simulink model "testemplanner_cs"  (R2023a)
settings: Solver=ode5  StartTime=0.0  StopTime=70  FixedStep=1/1000  RelTol=1e-3
PreLoadFcn:
  | mbxruntime.callbacks.PreLoadFcn(bdroot);
PostLoadFcn:
  | mbxruntime.callbacks.PostLoadFcn(bdroot);
InitFcn:
  | mbxruntime.callbacks.InitFcn(bdroot);
StartFcn:
  | mbxruntime.callbacks.StartFcn(bdroot);
StopFcn:
  | mbxruntime.callbacks.StopFcn(bdroot);
model workspace (MAT data in the model file):
  mbox_table : object (value not decoded)
  model_closed = 0
  sim_status = 0
values from neighbouring files (symbols this model uses):
  c_factor = 43.75    [emplanner_init.m]
  cf = -175016    [emplanner_init.m]
  cr = -130634    [emplanner_init.m]
  global_path_x = [-4.4795 -3.48011774493 -2.48199463442 -1.48514775065 -0.489582877207 0.504698358082 1.49769585569 2.48941007764 3.47984169183 4.46899144113 5.45686009523 6.44344843293 ... (3001 elements, 3001x1)]    [global_path.mat]
  global_path_y = [6.0531 6.0531 6.0531 6.0531 6.0531 6.0531 6.0531 6.0531 6.0531 6.0531 6.0531 6.0531 ... (3001 elements, 3001x1)]    [global_path.mat]
  KD_PID_distance = 0.0    (= 0)    [emplanner_init.m]
  KD_PID_speed = 0    [emplanner_init.m]
  KI_PID_distance = 0.0    (= 0)    [emplanner_init.m]
  KI_PID_speed = 0    [emplanner_init.m]
  KP_PID_distance = 0.5    [emplanner_init.m]
  KP_PID_speed = 1.8    [emplanner_init.m]
  la = 1.265    [emplanner_init.m]
  lb = 2.947-1.265    (= 1.682)    [emplanner_init.m]
  LQR_K1 = k(:,1)'    [emplanner_init.m]
  LQR_K2 = k(:,2)'    [emplanner_init.m]
  LQR_K3 = k(:,3)'    [emplanner_init.m]
  LQR_K4 = k(:,4)'    [emplanner_init.m]
  m = 2020    [emplanner_init.m]
  rack_displacement = [-39.14 , -37.2 , -35.29 , -33.43 , -31.6 , -29.81 , -28.06 , -26.34 , -24.66 ,      -23.01 , -21.38 , -19.79 , -18.23 , -16.69 , -15.18 , -13.7 , -12.23 , -10.8 , -9.38 , -7.98 ,     -6.61 , -5.25 , -3.91 , -2.59 , -1.29 , 0 , 1.27 , 2.54 , 3.78 , 5.02 , 6.24 , 7.46 , 8.66 ,      9.86 , 11.05 , 12.24 , 13.41 , 14.59 , 15.76 , 16.92 , 18.09 , 19.25 , 20.42 , 21.59 , 22.76 ,      23.93 , 25.11 , 26 ...(+26 chars)    [emplanner_init.m]
  right_wheel_ground = [-70 ,-67.2 , -64.4 , -61.6 , -58.8 , -56 , -53.2 , -50.4 , -47.6 , -44.8 , -42 ,      -39.2 , -36.4 , -33.6 , -30.8 , -28 , -25.2 , -22.4 , -19.6 , -16.8 , -14 , -11.2 , -8.4 , -5.6 ,      -2.8 , 0 , 2.8 , 5.6 , 8.4 , 11.2 , 14 , 16.8 , 19.6 , 22.4 , 25.2 , 28 , 30.8 , 33.6 , 36.4 ,      39.2 , 42 , 44.8 , 47.6 , 50.4 , 53.2 , 56 , 58.8 , 61.6 , 64.4 , 67.2 , 70 ]    [emplanner_init.m]
  vx_break_point = zeros(1,5000)    [emplanner_init.m]
undefined symbols (not defined in the file or in its folder): aubr, DiscIntNeverNeededParam, tablebr, vubr, warningInitialVelocity, x0
libraries: PreScanSimulinkLibrary x19, simulink x19, simulink_extras x6, Solver_SF x1
(part 4 of 10)

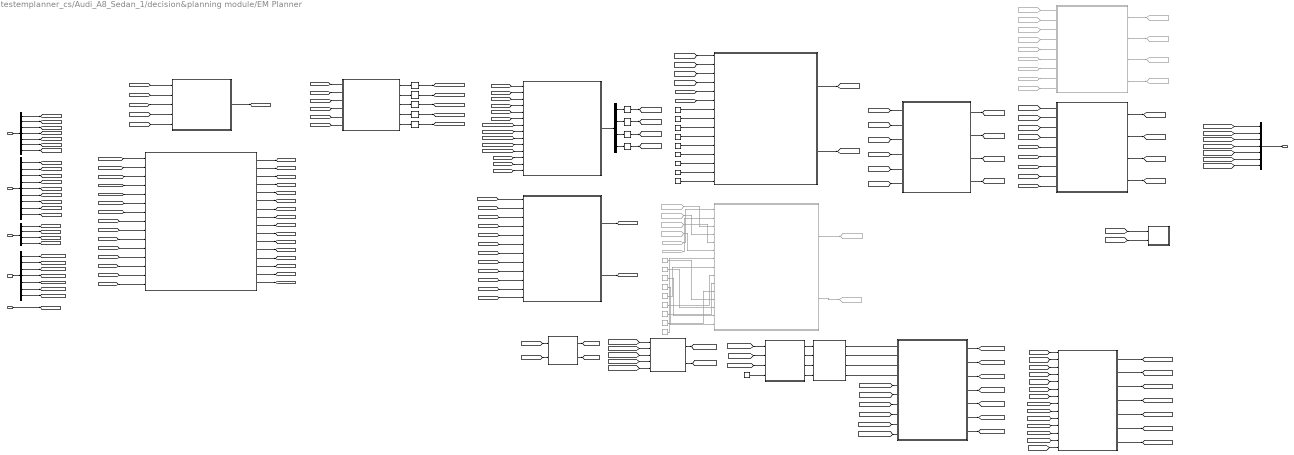
== system testemplanner_cs/Audi_A8_Sedan_1/decision&planning module/EM Planner ==
  referenceline_info : Inport
  location_info : Inport  Port=2
  perception_info : Inport  Port=3
  pre_planning_info : Inport  Port=4
  current time : Inport  Port=5
  Bus Creator : BusCreator  Inputs=7
  Bus Selector : BusSelector  OutputSignals=referenceline_x,referenceline_y,referenceline_heading,referenceline_kappa,origin_match_point_index,origin_proj_x,origin_proj_y
  Bus Selector1 : BusSelector  OutputSignals=host_x,host_y,host_heading_xy,host_vx,host_vy,host_yawrate,host_speed,host_ax,host_ay
  Bus Selector2 : BusSelector  OutputSignals=obs_x_set_gcs,obs_y_set_gcs,obs_velocity_set_gcs,obs_heading_set_gcs
  Bus Selector3 : BusSelector  OutputSignals=trajectory_x_gcs,trajectory_y_gcs,trajectory_heading_gcs,trajectory_kappa_gcs,trajectory_speed_gcs,trajectory_accel_gcs,trajectory_time_gcs
  Bus Selector4 : BusSelector  OutputSignals=s_set,l_set,dl_set,ddl_set
  Cartesian2Frenet-panning start point : Subsystem
  Constant : Constant  Value=9
  Constant1 : Constant  Value=4
  Constant10 : Constant  Commented=on  Value=9
  Constant11 : Constant  Commented=on  Value=4
  Constant12 : Constant  Commented=on  Value=15
  Constant13 : Constant  Commented=on
  Constant14 : Constant  Commented=on  Value=300
  Constant15 : Constant  Commented=on  Value=2000
  Constant16 : Constant  Commented=on  Value=10000
  Constant17 : Constant  Commented=on  Value=20
  Constant18 : Constant  Commented=on  Value=1e8
  Constant2 : Constant  Value=15
  Constant3 : Constant
  Constant4 : Constant  Value=300
  Constant5 : Constant  Value=2000
  Constant6 : Constant  Value=10000
  Constant7 : Constant  Value=20
  Constant8 : Constant  Value=1e8
  Constant9 : Constant  Value=8
  Dynamic Programming : MATLAB Function  TreatAsAtomicUnit=on
  Frenet2Cartesian : MATLAB Function  TreatAsAtomicUnit=on
  Frenet2Cartesian1 : MATLAB Function  Commented=on  TreatAsAtomicUnit=on
  From103 : From  Commented=on  GotoTag=planning_start_dl
  From109 : From  Commented=on  GotoTag=planning_start_ddl
  From116 : From  Commented=on  GotoTag=static_obs_s_set
  From117 : From  Commented=on  GotoTag=static_obs_l_set
  From118 : From  Commented=on  GotoTag=dp_path_s_final
  From119 : From  Commented=on  GotoTag=dp_path_l_final
  From120 : From  Commented=on  GotoTag=dp_path_dl_final
  From121 : From  Commented=on  GotoTag=dp_path_ddl_final
  From122 : From  Commented=on  GotoTag=referenceline_x
  From123 : From  Commented=on  GotoTag=referenceline_y
  From124 : From  Commented=on  GotoTag=referenceline_heading
  From125 : From  Commented=on  GotoTag=referenceline_kappa
  From126 : From  Commented=on  GotoTag=index2s
  From92 : From  Commented=on  GotoTag=planning_start_s
  From93 : From  Commented=on  GotoTag=planning_start_l
  Goto66 : Goto  Commented=on  GotoTag=dp_path_s_init
  Goto67 : Goto  Commented=on  GotoTag=dp_path_l_init
  Goto86 : Goto  Commented=on  GotoTag=trajectory_x_init
  Goto87 : Goto  Commented=on  GotoTag=trajectory_y_init
  Goto88 : Goto  Commented=on  GotoTag=trajectory_heading_init
  Goto89 : Goto  Commented=on  GotoTag=trajectory_kappa_init
  MATLAB Function : MATLAB Function  TreatAsAtomicUnit=on
  MATLAB Function1 : MATLAB Function  TreatAsAtomicUnit=on
  Obs : Subsystem
  Selector{1..9} (9 alike) : Selector  InputPortWidth=128  IndexOptions=Index vector (dialog)  Indices=1  OutputSizes=1
  cacul planning start gcs : MATLAB Function  TreatAsAtomicUnit=on
  calc path length and map between point and s : MATLAB Function  TreatAsAtomicUnit=on
  calc speed planning start condition : MATLAB Function  TreatAsAtomicUnit=on
  generate index2s : MATLAB Function  TreatAsAtomicUnit=on
  increase st point count : MATLAB Function  TreatAsAtomicUnit=on
  match&proj point search2 : MATLAB Function  TreatAsAtomicUnit=on
  path and speed merge : MATLAB Function  TreatAsAtomicUnit=on
  path decision with dynamic planning(dp) : MATLAB Function  Commented=on  TreatAsAtomicUnit=on
  simple speed qp planning : MATLAB Function  TreatAsAtomicUnit=on
  stitch trajectory : MATLAB Function  TreatAsAtomicUnit=on
  EM Planner result : Outport
  wires:
  referenceline_info/1 -> Bus Selector/1
  Bus Selector/1 -> [referenceline_x]  "<referenceline_x>"
  Bus Selector/2 -> [referenceline_y]  "<referenceline_y>"
  Bus Selector/3 -> [referenceline_heading]  "<referenceline_heading>"
  Bus Selector/4 -> [referenceline_kappa]  "<referenceline_kappa>"
  location_info/1 -> Bus Selector1/1
  Bus Selector1/1 -> [host_x]  "<host_x>"
  Bus Selector1/2 -> [host_y]  "<host_y>"
  Bus Selector1/3 -> [host_heading_xy]  "<host_heading_xy>"
  Bus Selector1/4 -> [host_vx_vcs]  "<host_vx>"
  Bus Selector1/5 -> [host_vy_vcs]  "<host_vy>"
  Bus Selector1/6 -> [host_yawrate]  "<host_yawrate>"
  Bus Selector1/7 -> [host_speed]  "<host_speed>"
  Bus Selector1/8 -> [host_ax_vcs]  "<host_ax>"
  Bus Selector1/9 -> [host_ay_vcs]  "<host_ay>"
  perception_info/1 -> Bus Selector2/1
  Bus Selector2/1 -> [obs_x_set_gcs]  "<obs_x_set_gcs>"
  Bus Selector2/2 -> [obs_y_set_gcs]  "<obs_y_set_gcs>"
  Bus Selector2/3 -> [obs_velocity_set_gcs]  "<obs_velocity_set_gcs>"
  Bus Selector2/4 -> [obs_heading_set_gcs]  "<obs_heading_set_gcs>"
  pre_planning_info/1 -> Bus Selector3/1
  Bus Selector3/1 -> [pre_trajectory_x_gcs]  "<trajectory_x_gcs>"
  Bus Selector3/2 -> [pre_trajectory_y_gcs]  "<trajectory_y_gcs>"
  Bus Selector3/3 -> [pre_trajectory_heading_gcs]  "<trajectory_heading_gcs>"
  Bus Selector3/4 -> [pre_trajectory_kappa_gcs]  "<trajectory_kappa_gcs>"
  Bus Selector3/5 -> [pre_trajectory_speed_gcs]  "<trajectory_speed_gcs>"
  Bus Selector3/6 -> [pre_trajectory_accel_gcs]  "<trajectory_accel_gcs>"
  current time/1 -> [current_time]
  [pre_trajectory_x_gcs] -> cacul planning start gcs/1(pre_trajectory_x)
  [pre_trajectory_y_gcs] -> cacul planning start gcs/2(pre_trajectory_y)
  [pre_trajectory_heading_gcs] -> cacul planning start gcs/3(pre_trajectory_heading)
  [pre_trajectory_kappa_gcs] -> cacul planning start gcs/4(pre_trajectory_kappa)
  [pre_trajectory_speed_gcs] -> cacul planning start gcs/5(pre_trajectory_speed)
  [pre_trajectory_accel_gcs] -> cacul planning start gcs/6(pre_trajectory_accel)
  [pre_trajectory_time] -> cacul planning start gcs/7(pre_trajectory_time)
  [current_time] -> cacul planning start gcs/8(current_time)
  [host_x] -> cacul planning start gcs/9(host_x)
  [host_y] -> cacul planning start gcs/10(host_y)
  [host_heading_xy] -> cacul planning start gcs/11(host_heading_xy)
  [host_vx_vcs] -> cacul planning start gcs/12(host_vx)
  [host_vy_vcs] -> cacul planning start gcs/13(host_vy)
  [host_ax_vcs] -> cacul planning start gcs/14(host_ax)
  [host_ay_vcs] -> cacul planning start gcs/15(host_ay)
  cacul planning start gcs/1(planning_start_x) -> [planning_start_x]
  cacul planning start gcs/2(planning_start_y) -> [planning_start_y]
  cacul planning start gcs/3(planning_start_heading) -> [planning_start_heading]
  cacul planning start gcs/4(planning_start_kappa) -> [planning_start_kappa]
  cacul planning start gcs/5(planning_start_vx) -> [planning_start_vx]
  cacul planning start gcs/6(planning_start_vy) -> [planning_start_vy]
  cacul planning start gcs/7(planning_start_ax) -> [planning_start_ax]
  cacul planning start gcs/8(planning_start_ay) -> [planning_start_ay]
  cacul planning start gcs/9(planning_start_time) -> [planning_start_time]
  cacul planning start gcs/10(stitch_x) -> [stitch_x]
  cacul planning start gcs/11(stitch_y) -> [stitch_y]
  cacul planning start gcs/12(stitch_heading) -> [stitch_heading]
  cacul planning start gcs/13(stitch_kappa) -> [stitch_kappa]
  cacul planning start gcs/14(stitch_speed) -> [stitch_speed]
  cacul planning start gcs/15(stitch_accel) -> [stitch_accel]
  cacul planning start gcs/16(stitch_time) -> [stitch_time]
  Bus Selector/5 -> [origin_match_point_index]  "<origin_match_point_index>"
  Bus Selector/6 -> [origin_proj_x]  "<origin_proj_x>"
  Bus Selector/7 -> [origin_proj_y]  "<origin_proj_y>"
  [origin_match_point_index] -> generate index2s/1(origin_match_point_index)
  [origin_proj_x] -> generate index2s/2(origin_proj_x)
  [origin_proj_y] -> generate index2s/3(origin_proj_y)
  [referenceline_x] -> generate index2s/4(path_x)
  [referenceline_y] -> generate index2s/5(path_y)
  generate index2s/1(index2s) -> [index2s]
  match&proj point search2/3(proj_y_set) -> Selector3/1
  match&proj point search2/1(match_point_index_set) -> Selector1/1
  match&proj point search2/2(proj_x_set) -> Selector2/1
  match&proj point search2/4(proj_heading_set) -> Selector4/1
  match&proj point search2/5(proj_kappa_set) -> Selector5/1
  [planning_start_x] -> match&proj point search2/1(x_set)
  [planning_start_y] -> match&proj point search2/2(y_set)
  [referenceline_x] -> match&proj point search2/3(frenet_x_set)
  [referenceline_y] -> match&proj point search2/4(frenet_y_set)
  [referenceline_heading] -> match&proj point search2/5(frenet_heading_set)
  [referenceline_kappa] -> match&proj point search2/6(frenet_kapppa_set)
  Selector1/1 -> [planning_start_match_point_index]
  Selector2/1 -> [planning_start_proj_x]
  Selector3/1 -> [planning_start_proj_y]
  Selector4/1 -> [planning_start_proj_heading]
  Selector5/1 -> [planning_start_proj_kappa]
  Cartesian2Frenet-panning start point/1(Caetesian2Frenetout) -> Bus Selector4/1
  Bus Selector4/1 -> Selector6/1  "<s_set>"
  Bus Selector4/2 -> Selector7/1  "<l_set>"
  Bus Selector4/3 -> Selector8/1  "<dl_set>"
  Bus Selector4/4 -> Selector9/1  "<ddl_set>"
  [planning_start_x] -> Cartesian2Frenet-panning start point/1(x_set)
  [planning_start_y] -> Cartesian2Frenet-panning start point/2(y_set)
  [planning_start_vx] -> Cartesian2Frenet-panning start point/3(vx_set)
  [planning_start_vy] -> Cartesian2Frenet-panning start point/4(vy_set)
  [planning_start_ax] -> Cartesian2Frenet-panning start point/5(ax_set)
  [planning_start_ay] -> Cartesian2Frenet-panning start point/6(ay_set)
  [planning_start_proj_x] -> Cartesian2Frenet-panning start point/7(proj_x_set)
  [planning_start_proj_y] -> Cartesian2Frenet-panning start point/8(proj_y_set)
  [planning_start_proj_heading] -> Cartesian2Frenet-panning start point/9(proj_heading_set)
  [planning_start_proj_kappa] -> Cartesian2Frenet-panning start point/10(proj_kappa_set)
  [planning_start_match_point_index] -> Cartesian2Frenet-panning start point/11(match_point_index_set)
  [referenceline_x] -> Cartesian2Frenet-panning start point/12(frenet_x_set)
  [referenceline_y] -> Cartesian2Frenet-panning start point/13(frenet_y_set)
  [index2s] -> Cartesian2Frenet-panning start point/14(index2s)
  Selector6/1 -> [planning_start_s]
  Selector7/1 -> [planning_start_l]
  Selector8/1 -> [planning_start_dl]
  Selector9/1 -> [planning_start_ddl]
  [host_x] -> Obs/1(host_x)
  [host_y] -> Obs/2(host_y)
  [obs_x_set_gcs] -> Obs/3(obs_x_set_gcs)
  [obs_y_set_gcs] -> Obs/4(obs_y_set_gcs)
  [obs_velocity_set_gcs] -> Obs/5(obs_velocity_set_gcs)
  [obs_heading_set_gcs] -> Obs/6(obs_heading_set_gcs)
  [host_heading_xy] -> Obs/7(host_heading_xy)
  [index2s] -> Obs/12(index2s)
  [referenceline_x] -> Obs/8(referenceline_x)
  [referenceline_y] -> Obs/9(referenceline_y)
  [referenceline_heading] -> Obs/10(referenceline_heading)
  [referenceline_kappa] -> Obs/11(referenceline_kappa)
  Obs/1(static_obs_s_set) -> [static_obs_s_set]
  Obs/2(static_obs_l_set) -> [static_obs_l_set]
  [planning_start_s] -> Dynamic Programming/1(planning_start_s)
  [planning_start_l] -> Dynamic Programming/2(planning_start_l)
  [planning_start_dl] -> Dynamic Programming/3(planning_start_dl)
  [planning_start_ddl] -> Dynamic Programming/4(planning_start_ddl)
  [static_obs_l_set] -> Dynamic Programming/6(obs_l_set)
  [static_obs_s_set] -> Dynamic Programming/5(obs_s_set)
  Constant/1 -> Dynamic Programming/7(row)
  Constant1/1 -> Dynamic Programming/8(col)
  Constant2/1 -> Dynamic Programming/9(sample_s)
  Constant3/1 -> Dynamic Programming/10(sample_l)
  Constant4/1 -> Dynamic Programming/11(w_dl_smooth_cost)
  Constant5/1 -> Dynamic Programming/12(w_ddl_smooth_cost)
  Constant6/1 -> Dynamic Programming/13(w_dddl_smooth_cost)
  Constant7/1 -> Dynamic Programming/14(w_reference_cost)
  Constant8/1 -> Dynamic Programming/15(w_collision_cost)
  Dynamic Programming/1(dp_path_s) -> [dp_path_s_init]
  Dynamic Programming/2(dp_path_l) -> [dp_path_l_init]
  [dp_path_s_init] -> MATLAB Function/1(dp_path_s_init)
  [dp_path_l_init] -> MATLAB Function/2(dp_path_l_init)
  [planning_start_s] -> MATLAB Function/3(plan_start_s)
  [planning_start_dl] -> MATLAB Function/5(plan_start_dl)
  [planning_start_ddl] -> MATLAB Function/6(plan_start_ddl)
  [planning_start_l] -> MATLAB Function/4(plan_start_l)
  MATLAB Function/1(dp_path_s_final) -> [dp_path_s_final]
  MATLAB Function/2(dp_path_l_final) -> [dp_path_l_final]
  MATLAB Function/3(dp_path_dl_final) -> [dp_path_dl_final]
  MATLAB Function/4(dp_path_ddl_final) -> [dp_path_ddl_final]
  [dp_path_s_final] -> Frenet2Cartesian/1(s_set)
  [dp_path_l_final] -> Frenet2Cartesian/2(l_set)
  [dp_path_dl_final] -> Frenet2Cartesian/3(dl_set)
  [dp_path_ddl_final] -> Frenet2Cartesian/4(ddl_set)
  [referenceline_x] -> Frenet2Cartesian/5(frenet_x)
  [referenceline_y] -> Frenet2Cartesian/6(frenet_y)
  [referenceline_heading] -> Frenet2Cartesian/7(frenet_heading)
  [index2s] -> Frenet2Cartesian/9(index2s)
  [referenceline_kappa] -> Frenet2Cartesian/8(frenet_kappa)
  Frenet2Cartesian/1(x_point_set) -> [trajectory_x_init]
  Frenet2Cartesian/2(y_point_set) -> [trajectory_y_init]
  Frenet2Cartesian/3(heading_point_set) -> [trajectory_heading_init]
  Frenet2Cartesian/4(kappa_point_set) -> [trajectory_kappa_init]
  stitch trajectory/6(trajectory_accel_final) -> [trajectory_accel_final]
  stitch trajectory/7(trajectory_time_final) -> [trajectory_time_final]
  [trajectory_heading] -> stitch trajectory/3(trajectory_heading)
  [planning_start_time] -> path and speed merge/5(current_time)
  increase st point count/2(s_dot) -> path and speed merge/2(s_dot)
  [plan_start_s_dot] -> simple speed qp planning/1(plan_start_s_dot)
  [trajectory_x_final] -> Bus Creator/1  "trajectory_x_gcs"
  [stitch_kappa] -> stitch trajectory/11(stitch_kappa)
  [trajectory_y_final] -> Bus Creator/2  "trajectory_y_gcs"
  simple speed qp planning/4(relative_time_init) -> increase st point count/4(relative_time_init)
  path and speed merge/5(trajectory_speed) -> [trajectory_speed]
  simple speed qp planning/3(s_dot2_init) -> increase st point count/3(s_dot2_init)
  increase st point count/4(relative_time) -> path and speed merge/4(relative_time)
  [plan_start_s_dot2] -> simple speed qp planning/2(plan_start_s_dot2)
  simple speed qp planning/1(s_init) -> increase st point count/1(s_init)
  [trajectory_heading_init] -> path and speed merge/9(trajectory_heading_init)
  path and speed merge/7(trajectory_time) -> [trajectory_time]
  [trajectory_x] -> stitch trajectory/1(trajectory_x)
  path and speed merge/6(trajectory_accel) -> [trajectory_accel]
  [stitch_speed] -> stitch trajectory/12(stitch_speed)
  [trajectory_y] -> stitch trajectory/2(trajectory_y)
  [stitch_accel] -> stitch trajectory/13(stitch_accel)
  stitch trajectory/3(trajectory_heading_final) -> [trajectory_heading_final]
  [trajectory_x_init] -> path and speed merge/7(trajectory_x_init)
  [path_s] -> path and speed merge/6(path_s)
  [path_s_end] -> simple speed qp planning/3(s_end)
  calc speed planning start condition/2(plan_start_s_dot2) -> [plan_start_s_dot2]
  stitch trajectory/5(trajectory_speed_final) -> [trajectory_speed_final]
  Constant9/1 -> simple speed qp planning/4(recommend_T)
  [trajectory_time] -> stitch trajectory/7(trajectory_time)
  [stitch_time] -> stitch trajectory/14(stitch_time)
  [planning_start_ay] -> calc speed planning start condition/4(plan_start_ay)
  [trajectory_accel] -> stitch trajectory/6(trajectory_accel)
  [stitch_heading] -> stitch trajectory/10(stitch_heading)
  [trajectory_kappa] -> stitch trajectory/4(trajectory_kappa)
  [trajectory_heading_final] -> Bus Creator/3  "trajectory_heading_gcs"
  [trajectory_speed_final] -> Bus Creator/5  "trajectory_speed_gcs"
  increase st point count/3(s_dot2) -> path and speed merge/3(s_dot2)
  calc path length and map between point and s/2(path_s) -> [path_s]
  [trajectory_time_final] -> Bus Creator/7  "trajectory_time_gcs"
  stitch trajectory/4(trajectory_kappa_final) -> [trajectory_kappa_final]
  calc path length and map between point and s/1(path_s_end) -> [path_s_end]
  [planning_start_vy] -> calc speed planning start condition/2(plan_start_vy)
  increase st point count/1(s) -> path and speed merge/1(s)
  [planning_start_heading] -> calc speed planning start condition/5(plan_start_heading)
  [trajectory_accel_final] -> Bus Creator/6  "trajectory_accel_gcs"
  path and speed merge/4(trajectory_kappa) -> [trajectory_kappa]
  [stitch_y] -> stitch trajectory/9(stitch_y)
  path and speed merge/1(trajectory_x) -> [trajectory_x]
  stitch trajectory/1(trajectory_x_final) -> [trajectory_x_final]
  [trajectory_x_init] -> calc path length and map between point and s/1(trajectory_x)
  stitch trajectory/2(trajectory_y_final) -> [trajectory_y_final]
  calc speed planning start condition/1(plan_start_s_dot) -> [plan_start_s_dot]
  [trajectory_y_init] -> calc path length and map between point and s/2(trajectory_y)
  [trajectory_speed] -> stitch trajectory/5(trajectory_speed)
  [trajectory_kappa_init] -> path and speed merge/10(trajectory_kappa_init)
  [planning_start_vx] -> calc speed planning start condition/1(plan_start_vx)
  [trajectory_y_init] -> path and speed merge/8(trajectory_y_init)
  path and speed merge/2(trajectory_y) -> [trajectory_y]
  path and speed merge/3(trajectory_heading) -> [trajectory_heading]
  Bus Creator/1 -> EM Planner result/1
  [stitch_x] -> stitch trajectory/8(stitch_x)
  simple speed qp planning/2(s_dot_init) -> increase st point count/2(s_dot_init)
  [planning_start_ax] -> calc speed planning start condition/3(plan_start_ax)
  [trajectory_kappa_final] -> Bus Creator/4  "trajectory_kappa_gcs"
  Bus Selector3/7 -> [pre_trajectory_time]  "<trajectory_time_gcs>"
  [dp_path_s_final] -> MATLAB Function1/1(s)
  [dp_path_l_final] -> MATLAB Function1/2(l)
  path decision with dynamic planning(dp)/2(dp_path_l) -> Goto67/1
  path decision with dynamic planning(dp)/1(dp_path_s) -> Goto66/1
  Constant18/1 -> path decision with dynamic planning(dp)/7(w_cost_collision)
  Constant17/1 -> path decision with dynamic planning(dp)/11(w_cost_ref)
  Constant16/1 -> path decision with dynamic planning(dp)/10(w_cost_smooth_dddl)
  Constant15/1 -> path decision with dynamic planning(dp)/9(w_cost_smooth_ddl)
  Constant14/1 -> path decision with dynamic planning(dp)/8(w_cost_smooth_dl)
  Constant13/1 -> path decision with dynamic planning(dp)/15(sample_l)
  Constant12/1 -> path decision with dynamic planning(dp)/14(sample_s)
  Constant11/1 -> path decision with dynamic planning(dp)/13(col)
  Constant10/1 -> path decision with dynamic planning(dp)/12(row)
  From116/1 -> path decision with dynamic planning(dp)/1(obs_s_set)
  From117/1 -> path decision with dynamic planning(dp)/2(obs_l_set)
  From109/1 -> path decision with dynamic planning(dp)/6(plan_start_dll)
  From103/1 -> path decision with dynamic planning(dp)/5(plan_start_dl)
  From93/1 -> path decision with dynamic planning(dp)/4(plan_start_l)
  From92/1 -> path decision with dynamic planning(dp)/3(plan_start_s)
  Frenet2Cartesian1/4(kappa_set) -> Goto89/1
  Frenet2Cartesian1/3(heading_set) -> Goto88/1
  Frenet2Cartesian1/2(y_set) -> Goto87/1
  Frenet2Cartesian1/1(x_set) -> Goto86/1
  From125/1 -> Frenet2Cartesian1/8(frenet_path_kappa)
  From126/1 -> Frenet2Cartesian1/9(index2s)
  From124/1 -> Frenet2Cartesian1/7(frenet_path_heading)
  From123/1 -> Frenet2Cartesian1/6(frenet_path_y)
  From122/1 -> Frenet2Cartesian1/5(frenet_path_x)
  From121/1 -> Frenet2Cartesian1/4(ddl_set)
  From120/1 -> Frenet2Cartesian1/3(dl_set)
  From119/1 -> Frenet2Cartesian1/2(l_set)
  From118/1 -> Frenet2Cartesian1/1(s_set)

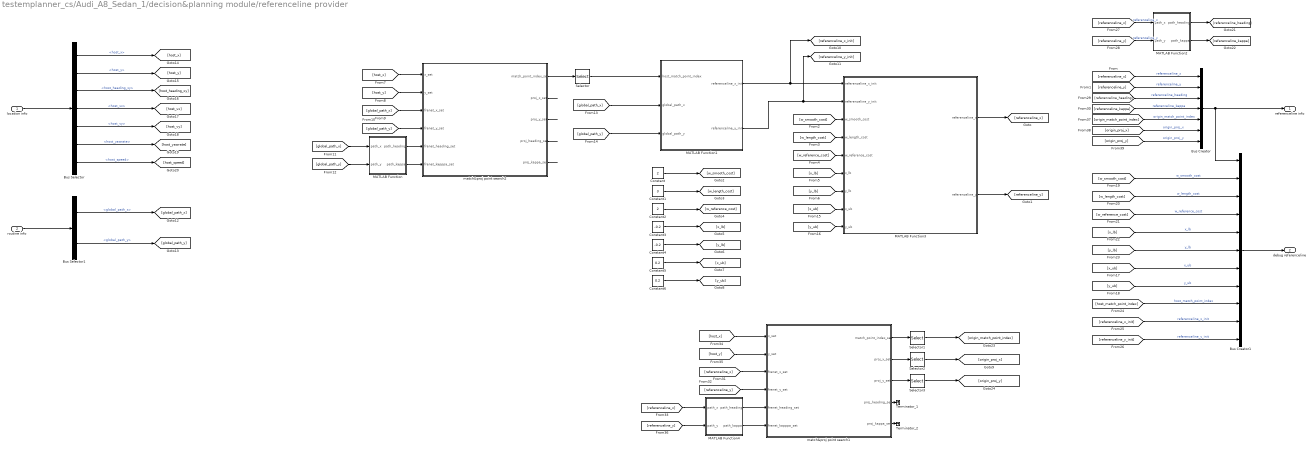
== system testemplanner_cs/Audi_A8_Sedan_1/decision&planning module/referenceline provider ==
  location info : Inport
  routine info : Inport  Port=2
  Bus Creator : BusCreator  Inputs=7
  Bus Creator1 : BusCreator  Inputs=11
  Bus Selector : BusSelector  OutputSignals=host_x,host_y,host_heading_xy,host_vx,host_vy,host_yawrate,host_speed
  Bus Selector1 : BusSelector  OutputSignals=global_path_x,global_path_y
  Constant : Constant  Value=2
  Constant1 : Constant  Value=3
  Constant2 : Constant  Value=2
  Constant3 : Constant  Value=-0.2
  Constant4 : Constant  Value=-0.2
  Constant5 : Constant  Value=0.2
  Constant6 : Constant  Value=0.2
  MATLAB Function : MATLAB Function  TreatAsAtomicUnit=on
  MATLAB Function1 : MATLAB Function  TreatAsAtomicUnit=on
  MATLAB Function2 : MATLAB Function  TreatAsAtomicUnit=on
  MATLAB Function3 : MATLAB Function  TreatAsAtomicUnit=on
  MATLAB Function4 : MATLAB Function  TreatAsAtomicUnit=on
  Selector{,1..3} (4 alike) : Selector  InputPortWidth=128  IndexOptions=Index vector (dialog)  Indices=1  OutputSizes=1
  Terminator_1 : Terminator
  Terminator_2 : Terminator
  match&proj point search1 : MATLAB Function  TreatAsAtomicUnit=on
  match&proj point search2 : MATLAB Function  TreatAsAtomicUnit=on
  referenceline info : Outport
  debug referenceline : Outport  Port=2
  wires:
  [x_lb] -> MATLAB Function3/6(x_lb)
  [global_path_x] -> MATLAB Function/1(path_x)
  [global_path_x] -> match&proj point search2/3(frenet_x_set)
  [w_reference_cost] -> MATLAB Function3/5(w_reference_cost)
  MATLAB Function1/1(referenceline_x_init) -> [referenceline_x_init], MATLAB Function3/1(referenceline_x_init)
  [w_smooth_cost] -> MATLAB Function3/3(w_smooth_cost)
  [host_y] -> match&proj point search2/2(y_set)
  match&proj point search2/1(match_point_index_set) -> Selector/1
  [global_path_y] -> MATLAB Function/2(path_y)
  MATLAB Function/2(path_kappa) -> match&proj point search2/6(frenet_kapppa_set)
  Constant4/1 -> [y_lb]
  [global_path_x] -> MATLAB Function1/2(global_path_x)
  MATLAB Function/1(path_heading) -> match&proj point search2/5(frenet_heading_set)
  [global_path_y] -> MATLAB Function1/3(global_path_y)
  Selector/1 -> MATLAB Function1/1(host_match_point_index)
  Constant2/1 -> [w_reference_cost]
  [global_path_y] -> match&proj point search2/4(frenet_y_set)
  [host_x] -> match&proj point search2/1(x_set)
  [w_length_cost] -> MATLAB Function3/4(w_length_cost)
  MATLAB Function1/2(referenceline_y_init) -> [referenceline_y_init], MATLAB Function3/2(referenceline_y_init)
  Constant/1 -> [w_smooth_cost]
  Constant1/1 -> [w_length_cost]
  Constant3/1 -> [x_lb]
  [x_ub] -> MATLAB Function3/8(x_ub)
  [y_lb] -> MATLAB Function3/7(y_lb)
  [y_ub] -> MATLAB Function3/9(y_ub)
  Constant6/1 -> [y_ub]
  Constant5/1 -> [x_ub]
  MATLAB Function3/1(referenceline_x) -> [referenceline_x]
  MATLAB Function3/2(referenceline_y) -> [referenceline_y]
  Bus Creator/1 -> Bus Creator1/1, referenceline info/1
  [referenceline_y] -> Bus Creator/2  "referenceline_y"
  [referenceline_x] -> Bus Creator/1  "referenceline_x"
  Bus Creator1/1 -> debug referenceline/1
  [w_smooth_cost] -> Bus Creator1/2  "w_smooth_cost"
  [w_length_cost] -> Bus Creator1/3  "w_length_cost"
  [w_reference_cost] -> Bus Creator1/4  "w_reference_cost"
  [x_lb] -> Bus Creator1/5  "x_lb"
  [y_lb] -> Bus Creator1/6  "y_lb"
  [x_ub] -> Bus Creator1/7  "x_ub"
  [y_ub] -> Bus Creator1/8  "y_ub"
  [host_match_point_index] -> Bus Creator1/9  "host_match_point_index"
  [referenceline_x_init] -> Bus Creator1/10  "referenceline_x_init"
  [referenceline_y_init] -> Bus Creator1/11  "referenceline_y_init"
  Bus Selector1/2 -> [global_path_y]  "<global_path_y>"
  Bus Selector1/1 -> [global_path_x]  "<global_path_x>"
  routine info/1 -> Bus Selector1/1
  Bus Selector/7 -> [host_speed]  "<host_speed>"
  Bus Selector/6 -> [host_yawrate]  "<host_yawrate>"
  Bus Selector/2 -> [host_y]  "<host_y>"
  Bus Selector/1 -> [host_x]  "<host_x>"
  Bus Selector/3 -> [host_heading_xy]  "<host_heading_xy>"
  Bus Selector/4 -> [host_vx]  "<host_vx>"
  Bus Selector/5 -> [host_vy]  "<host_vy>"
  location info/1 -> Bus Selector/1
  [referenceline_y] -> MATLAB Function2/2(path_y)  "referenceline_y"
  [referenceline_x] -> MATLAB Function2/1(path_x)  "referenceline_x"
  MATLAB Function2/1(path_heading) -> [referenceline_heading]
  MATLAB Function2/2(path_kappa) -> [referenceline_kappa]
  [referenceline_heading] -> Bus Creator/3  "referenceline_heading"
  [referenceline_kappa] -> Bus Creator/4  "referenceline_kappa"
  [host_x] -> match&proj point search1/1(x_set)
  [referenceline_y] -> match&proj point search1/4(frenet_y_set)
  MATLAB Function4/1(path_heading) -> match&proj point search1/5(frenet_heading_set)
  MATLAB Function4/2(path_kappa) -> match&proj point search1/6(frenet_kapppa_set)
  [referenceline_y] -> MATLAB Function4/2(path_y)
  [host_y] -> match&proj point search1/2(y_set)
  [referenceline_x] -> match&proj point search1/3(frenet_x_set)
  [referenceline_x] -> MATLAB Function4/1(path_x)
  match&proj point search1/1(match_point_index_set) -> Selector1/1
  Selector1/1 -> [origin_match_point_index]
  match&proj point search1/2(proj_x_set) -> Selector2/1
  Selector2/1 -> [origin_proj_x]
  match&proj point search1/3(proj_y_set) -> Selector3/1
  Selector3/1 -> [origin_proj_y]
  [origin_match_point_index] -> Bus Creator/5  "origin_match_point_index"
  [origin_proj_x] -> Bus Creator/6  "origin_proj_x"
  [origin_proj_y] -> Bus Creator/7  "origin_proj_y"
  match&proj point search2/2(proj_x_set) -> ?
  match&proj point search2/3(proj_y_set) -> ?
  match&proj point search2/4(proj_heading_set) -> ?
  match&proj point search2/5(proj_kappa_set) -> ?
  match&proj point search1/4(proj_heading_set) -> Terminator_1/1
  match&proj point search1/5(proj_kappa_set) -> Terminator_2/1

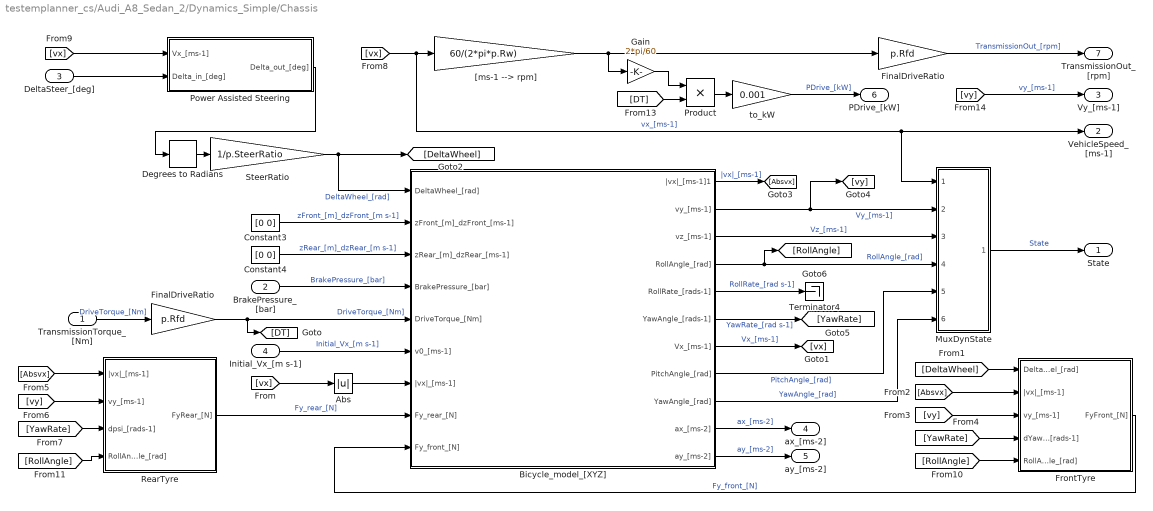
== system testemplanner_cs/Audi_A8_Sedan_2/Dynamics_Simple/Chassis ==
  TransmissionTorque_[Nm] : Inport
  BrakePressure_[bar] : Inport  Port=2
  DeltaSteer_[deg] : Inport  Port=3
  Initial_Vx_[m s-1] : Inport  Port=4
  Abs : Abs  SaturateOnIntegerOverflow=off
  Bicycle_model_[XYZ] : Subsystem
      mask Display: image(imread('Bicycle_model.png'));
  Constant3 : Constant  Value=[0 0]
  Constant4 : Constant  Value=[0 0]
  Degrees to Radians : simulink_extras/Transformations/Degrees to Radians
  FinalDriveRatio : Gain  Gain=p.Rfd  SaturateOnIntegerOverflow=on  OutDataTypeStr=Inherit: Same as input  ParamDataTypeStr=Inherit: Same as input
  "FinalDriveRatio " : Gain  Gain=p.Rfd  SaturateOnIntegerOverflow=on  OutDataTypeStr=Inherit: Same as input  ParamDataTypeStr=Inherit: Same as input
  FrontTyre : Subsystem
      mask Display: image(imread('Tyre.png'));
  Gain : Gain  Gain=2*pi/60
  MuxDynState : Subsystem
  Power Assisted Steering : Subsystem
  Product : Product  RndMeth=Zero
  RearTyre : Subsystem
      mask Display: image(imread('Tyre.png'));
  SteerRatio : Gain  Gain=1/p.SteerRatio
  Terminator4 : Terminator
  "[ms-1 --> rpm]" : Gain  Gain=60/(2*pi*p.Rw)  SaturateOnIntegerOverflow=on  OutDataTypeStr=Inherit: Same as input  ParamDataTypeStr=Inherit: Same as input
  to_kW : Gain  Gain=0.001
  State : Outport
  VehicleSpeed_[ms-1] : Outport  Port=2
  Vy_[ms-1] : Outport  Port=3
  ax_[ms-2] : Outport  Port=4
  ay_[ms-2] : Outport  Port=5
  PDrive_[kW] : Outport  Port=6
  TransmissionOut_[rpm] : Outport  Port=7
  wires:
  [vy] -> Vy_[ms-1]/1  "vy_[ms-1]"
  to_kW/1 -> PDrive_[kW]/1  "PDrive_[kW]"
  Gain/1 -> Product/1
  Bicycle_model_[XYZ]/10(ax_[ms-2]) -> ax_[ms-2]/1  "ax_[ms-2]"
  Product/1 -> to_kW/1
  [DT] -> Product/2
  Bicycle_model_[XYZ]/11(ay_[ms-2]) -> ay_[ms-2]/1  "ay_[ms-2]"
  Abs/1 -> Bicycle_model_[XYZ]/7(|vx|_[ms-1])
  Degrees to Radians/1 -> SteerRatio/1
  [vx] -> Abs/1
  SteerRatio/1 -> [DeltaWheel], Bicycle_model_[XYZ]/1(DeltaWheel_[rad])  "DeltaWheel_[rad]"
  TransmissionTorque_[Nm]/1 -> "FinalDriveRatio "/1  "DriveTorque_[Nm]"
  RearTyre/1(FyRear_[N]) -> Bicycle_model_[XYZ]/8(Fy_rear_[N])  "Fy_rear_[N]"
  FrontTyre/1(FyFront_[N]) -> Bicycle_model_[XYZ]/9(Fy_front_[N])  "Fy_front_[N]"
  Bicycle_model_[XYZ]/1(|vx|_[ms-1]1) -> [Absvx]  "|vx|_[ms-1]"
  Bicycle_model_[XYZ]/2(vy_[ms-1]) -> [vy], MuxDynState/2(vy [ms-1])  "Vy_[ms-1]"
  Bicycle_model_[XYZ]/4(RollAngle_[rad]) -> MuxDynState/4(R [rad]), [RollAngle]  "RollAngle_[rad]"
  Bicycle_model_[XYZ]/6(YawAngle_[rads-1]) -> [YawRate]  "YawRate_[rad s-1]"
  Bicycle_model_[XYZ]/7(Vx_[ms-1]) -> [vx]  "Vx_[ms-1]"
  [DeltaWheel] -> FrontTyre/1(DeltaWheel_[rad])
  [Absvx] -> FrontTyre/2(|vx|_[ms-1])
  [vy] -> FrontTyre/3(vy_[ms-1])
  [YawRate] -> FrontTyre/4(dYawAngle_[rads-1])
  [Absvx] -> RearTyre/1(|vx|_[ms-1])
  [vy] -> RearTyre/2(vy_[ms-1])
  [YawRate] -> RearTyre/3(dpsi_[rads-1])
  Bicycle_model_[XYZ]/3(vz_[ms-1]) -> MuxDynState/3(vz [ms-1])  "Vz_[ms-1]"
  Bicycle_model_[XYZ]/8(PitchAngle_[rad]) -> MuxDynState/5(P [rad])  "PitchAngle_[rad]"
  Bicycle_model_[XYZ]/9(YawAngle_[rad]) -> MuxDynState/6(Y [rad])  "YawAngle_[rad]"
  "[ms-1 --> rpm]"/1 -> Gain/1, FinalDriveRatio/1
  FinalDriveRatio/1 -> TransmissionOut_[rpm]/1  "TransmissionOut_[rpm]"
  [vx] -> "[ms-1 --> rpm]"/1, VehicleSpeed_[ms-1]/1, MuxDynState/1(vx [ms-1])  "vx_[ms-1]"
  [vx] -> Power Assisted Steering/1(Vx_[ms-1])
  DeltaSteer_[deg]/1 -> Power Assisted Steering/2(Delta_in_[deg])
  Power Assisted Steering/1(Delta_out_[deg]) -> Degrees to Radians/1
  [RollAngle] -> FrontTyre/5(RollAngle_[rad])
  [RollAngle] -> RearTyre/4(RollAngle_[rad])
  Constant3/1 -> Bicycle_model_[XYZ]/2(zFront_[m]_dzFront_[ms-1])  "zFront_[m]_dzFront_[m s-1]"
  Constant4/1 -> Bicycle_model_[XYZ]/3(zRear_[m]_dzRear_[ms-1])  "zRear_[m]_dzRear_[m s-1]"
  BrakePressure_[bar]/1 -> Bicycle_model_[XYZ]/4(BrakePressure_[bar])  "BrakePressure_[bar]"
  "FinalDriveRatio "/1 -> Bicycle_model_[XYZ]/5(DriveTorque_[Nm]), [DT]  "DriveTorque_[Nm]"
  Initial_Vx_[m s-1]/1 -> Bicycle_model_[XYZ]/6(v0_[ms-1])  "Initial_Vx_[m s-1]"
  Bicycle_model_[XYZ]/5(RollRate_[rads-1]) -> Terminator4/1  "RollRate_[rad s-1]"
  MuxDynState/1(State) -> State/1  "State"

== system testemplanner_cs/Audi_A8_Sedan_2/Dynamics_Simple/Engine ==
  ImpellerTorque_[Nm] : Inport
  Throttle_[%] : Inport  Port=2
  Configurable Subsystem : Subsystem  BlockChoice=Rate Limiter  mask{ComputationMode=ComputationMode}
      mask prompts: ComputationMode "Compuation mode:"
      mask init:
      | SetComputationMode(gcb,ComputationMode);
      settings: AttributesFormatString=%<BlockChoice>  OpenFcn=BringToFront(gcb);  MemberBlocks=Discrete Rate Limiter,Rate Limiter
      settings: TemplateBlock=|
      | PreScanSimulinkLibrary/Configurable Subsystems/TransferFunction
      | Engine/Configurable
      | Subsystem
  Configurable Subsystem1 : Subsystem  BlockChoice=Integrator  mask{ComputationMode=ComputationMode}
      mask prompts: ComputationMode "Computation mode:"
      mask init:
      | SetComputationMode(gcb,ComputationMode);
      settings: AttributesFormatString=%<BlockChoice>  OpenFcn=BringToFront(gcb);  MemberBlocks=Discrete-Time Integrator,Integrator
      settings: TemplateBlock=|
      | PreScanSimulinkLibrary/Configurable Subsystems/integral with initial condition and limts
      | for engine/Configurable
      | Subsystem
  EngineTorque : Lookup2D  RowIndex=p.thvec  ColumnIndex=p.nevec  Table=p.emap  SaturateOnIntegerOverflow=off
  Gain : Gain  Gain=2*pi/60
  Product : Product  RndMeth=Zero
  Sum : Sum  Inputs=-+  InputSameDT=on  SaturateOnIntegerOverflow=on  OutDataTypeStr=Inherit: Same as first input
  engine + impeller inertia : Gain  Gain=1/p.Iei  SaturateOnIntegerOverflow=on  OutDataTypeStr=Inherit: Same as input  ParamDataTypeStr=Inherit: Same as input
  rad|sec2rpm : Gain  Gain=60/2/pi  SaturateOnIntegerOverflow=on  OutDataTypeStr=Inherit: Same as input  ParamDataTypeStr=Inherit: Same as input
  to_kW : Gain  Gain=0.001
  nEngine_[rpm] : Outport  InitialOutput=0
  PEngine_[kW] : Outport  Port=2  InitialOutput=0
  wires:
  rad|sec2rpm/1 -> nEngine_[rpm]/1, EngineTorque/2, Gain/1  "rpm"
  engine + impeller inertia/1 -> Configurable Subsystem1/1(In1)  "rads-2"
  EngineTorque/1 -> Sum/2, Product/2
  Sum/1 -> engine + impeller inertia/1
  Configurable Subsystem1/1(Out1) -> rad|sec2rpm/1  "rads-1"
  Throttle_[%]/1 -> Configurable Subsystem/1(In1)
  ImpellerTorque_[Nm]/1 -> Sum/1
  Configurable Subsystem/1(Out1) -> EngineTorque/1
  Product/1 -> to_kW/1
  Gain/1 -> Product/1
  to_kW/1 -> PEngine_[kW]/1

== system testemplanner_cs/Audi_A8_Sedan_2/Dynamics_Simple/Gear: Auto Manual ==
  note: 0; Auto = on // Manual =off
      | 1; Auto = off // Manual =on
  Auto_Manual : Inport
  Manual_Gear : Inport  Port=2
  Auto_Gear : Inport  Port=3
  If : If  IfExpression=u1 == 0
  If Action Subsystem : Subsystem  TreatAsAtomicUnit=on
  If Action Subsystem1 : Subsystem  TreatAsAtomicUnit=on
  Merge : Merge
  Gear : Outport
  wires:
  If Action Subsystem/1(Out1) -> Merge/1
  Auto_Gear/1 -> If Action Subsystem/1(In1)
  If/1 -> If Action Subsystem/Action
  Merge/1 -> Gear/1
  If Action Subsystem1/1(Out1) -> Merge/2
  Manual_Gear/1 -> If Action Subsystem1/1(In1)
  If/2 -> If Action Subsystem1/Action
  Auto_Manual/1 -> If/1

== system testemplanner_cs/Audi_A8_Sedan_2/Dynamics_Simple/ShiftLogic ==
  Throttle_[%] : Inport
  GearNr_[-] : Inport  Port=2
  Auto_GearShift : Inport  Port=3
  VehSpeed_[ms-1] : Inport  Port=4
  Add2 : Sum
  Data Type Conversion1 : DataTypeConversion  OutDataTypeStr=double  SaturateOnIntegerOverflow=off  RndMeth=Floor
  Detect Increase1 : simulink/Logic and Bit Operations/Detect Increase  vinit=0.0  OutDataTypeStr=uint8
  Detect Increase : Subsystem
  Gear limitation : Saturate  UpperLimit=p.maxGear  LowerLimit=1
  Gear limitation while shifting : Saturate  UpperLimit=p.maxGear  LowerLimit=1
  GearNeutral : Constant  Value=0
  GearReverse : Constant  Value=-1
  "IC, gear = 1" : Memory  InitialCondition=1  InheritSampleTime=on
  If Action Neutral : Subsystem  TreatAsAtomicUnit=on
  If Action Normal : Subsystem  TreatAsAtomicUnit=on
  If Action Reverse : Subsystem  TreatAsAtomicUnit=on
  Memory : Memory  InheritSampleTime=on
  Merge : Merge  Inputs=3
  Relational Operator : RelationalOperator  OutDataTypeStr=boolean  InputSameDT=off
  Relational Operator1 : RelationalOperator  Operator=<=  OutDataTypeStr=boolean  InputSameDT=off
  Shift_Down time : Delay  DelayLength=p.ShiftDown_fac
  Shift_Up time : Delay  DelayLength=p.ShiftUp_fac
  Sum : Sum  Inputs=+-
  interp_down : Lookup2D  RowIndex=p.downth  ColumnIndex=[1:p.maxGear]  Table=p.downtab  LookUpMeth=Interpolation-Use End Values  SaturateOnIntegerOverflow=off
  interp_up : Lookup2D  RowIndex=p.upth  ColumnIndex=[1:p.maxGear]  Table=p.uptab  LookUpMeth=Interpolation-Use End Values  SaturateOnIntegerOverflow=off
  reverse/neutral/normal gear : If  IfExpression=u1 == 0  ElseIfExpressions=u1 < 0
  to_ms-1 : Gain  Gain=1/3.6
  "to_ms-1 " : Gain  Gain=1/3.6
  GearNr : Outport
  wires:
  Auto_GearShift/1 -> reverse/neutral/normal gear/1
  "IC, gear = 1"/1 -> If Action Normal/1(In1)
  Merge/1 -> GearNr/1
  If Action Reverse/1(Out1) -> Merge/2
  If Action Neutral/1(Out1) -> Merge/1
  If Action Normal/1(Out1) -> Merge/3
  reverse/neutral/normal gear/3 -> If Action Normal/Action
  reverse/neutral/normal gear/1 -> If Action Neutral/Action
  reverse/neutral/normal gear/2 -> If Action Reverse/Action
  GearReverse/1 -> If Action Reverse/1(In1)
  GearNeutral/1 -> If Action Neutral/1(In1)
  Shift_Down time/1 -> Sum/2
  Shift_Up time/1 -> Sum/1
  Detect Increase/1(Out1) -> Shift_Up time/1
  Data Type Conversion1/1 -> Shift_Down time/1
  Detect Increase1/1 -> Data Type Conversion1/1
  Sum/1 -> Add2/1
  Memory/1 -> Add2/2  "GearNr_[-]"
  Add2/1 -> Gear limitation while shifting/1
  Gear limitation while shifting/1 -> "IC, gear = 1"/1, Memory/1  "GearNr_[-]"
  Throttle_[%]/1 -> interp_down/1, interp_up/1
  Relational Operator/1 -> Detect Increase/2(In2)
  Relational Operator1/1 -> Detect Increase1/1
  interp_down/1 -> "to_ms-1 "/1
  VehSpeed_[ms-1]/1 -> Relational Operator/1, Relational Operator1/1
  interp_up/1 -> to_ms-1/1
  Gear limitation/1 -> interp_down/2, interp_up/2, Detect Increase/1(GearNr_[-])
  GearNr_[-]/1 -> Gear limitation/1
  to_ms-1/1 -> Relational Operator/2
  "to_ms-1 "/1 -> Relational Operator1/2

== system testemplanner_cs/Audi_A8_Sedan_2/Dynamics_Simple/Transmission ==
  nEngine_[rpm] : Inport
  GearNr_[-] : Inport  Port=2
  n_TransmissionOut_[rpm] : Inport  Port=3
  Torque_Converter : Subsystem
      mask Display: image(imread('TorqueConverter.png'));
  Transmission_Ratio : Subsystem
  Viscous coupling : Lookup  InputValues=[-5:0.1:5]*p.m/4  Table=p.m/4*tanh([-5:0.1:5])  SaturateOnIntegerOverflow=off
  ImpellerTorque_[Nm] : Outport  InitialOutput=0
  TransmissionTorque_[Nm] : Outport  Port=2  InitialOutput=0
  wires:
  Torque_Converter/2(TurbineTorque_[Nm]) -> Viscous coupling/1  "Converter_Torque_[Nm]"
  Transmission_Ratio/2(nTransmissionIn_[rpm]) -> Torque_Converter/2(nTransmission_[rpm])
  nEngine_[rpm]/1 -> Torque_Converter/1(nEngine_[rpm])
  GearNr_[-]/1 -> Transmission_Ratio/2(GearNr_[-]), Torque_Converter/3(Gear nr)
  n_TransmissionOut_[rpm]/1 -> Transmission_Ratio/3(nTransmissionOut_[rpm])
  Torque_Converter/1(ImpellerTorque_[Nm]) -> ImpellerTorque_[Nm]/1
  Transmission_Ratio/1(tTransmissionOut_[Nm]) -> TransmissionTorque_[Nm]/1
  Viscous coupling/1 -> Transmission_Ratio/1(tTransmissionIn_[Nm])

== system testemplanner_cs/Audi_A8_Sedan_2/PathFollower_Preview_1/LateralController ==
  TrajOffset x,y,Y [m,m,deg] : Inport
  ActorOffset_Left(+) / Right(-) [m] : Inport  Port=2
  position x,y,Y [m,m,deg] : Inport  Port=3
  vx [m/s] : Inport  Port=4
  vy [m/s] : Inport  Port=5
  Yaw rate [deg/s] : Inport  Port=6
  CorneringStiffness_Tyres_Front [N/rad] : Inport  Port=7
  CorneringStiffness_Tyres_Rear [N/rad] : Inport  Port=8
  steering_ratio[-] : Inport  Port=9
  Avoid_0 : Saturate  UpperLimit=1000  LowerLimit=0.1
  CTRL REFERENCES : Subsystem
  Calculate delta steering error : Subsystem
      mask Display:
      | port_label('input', 1, 'v_x_vehicle [m/s]')
      | port_label('input', 2, 'v_x_vehicle_Min [m/s]')
      | port_label('input', 3, 't_Preview_LatCtrl [s]')
      | port_label('input', 4, 'v_y_vehicle [m/s]')
      | port_label('input', 5, 'yawrate_vehicle [rad/sec]')
      | port_label('input', 6, 'CorneringStiffness_Tyres_Front [N/rad]')
      | port_label('input', 7, 'CorneringStiffness_Tyres_Rear [N/rad]')
      | port_label('input', 8, 'm_vehicle_total [kg]')
      | port_label('input', 9, 'inertia_z_vehicle_total [kg m2]')
      | port_label('input', 10, 'e_Lat [m]')
      | port_label('input', 11, 'Distance_frontaxle_COG(+) [m]')
      | port_label('input', 12, 'wheel_base [m]')
      | port_label('output', 1, 'delta_steeringwheel [rad]')
  Const_t_Preview_LatCtrl[s] : Constant  Value=PreviewTime  SampleTime=CSSampleTime
  Const_v_x_Vehicle_Min[km|h] : Constant  Value=LowSpeedLimit  SampleTime=CSSampleTime
  Constant6 : Constant  SampleTime=CSSampleTime
  Demux : Demux  Outputs=3
  Demux1 : Demux  Outputs=3
  Distance_frontaxle_COG(+) [m] : Constant  Value=length_a  SampleTime=CSSampleTime
  Gain : Gain  Gain=1*pi/180
  Gain1 : Gain  Gain=1*pi/180
  Gain4 : Gain
  Memory : Memory  InheritSampleTime=on
  Memory1 : Memory  InheritSampleTime=on
  Memory2 : Memory  InheritSampleTime=on
  Mux : Mux  Inputs=3
  Mux1 : Mux  Inputs=3
  SteeringWheelAngle : Subsystem
  deg to rad : Gain  Gain=pi/180
  inertia_z_vehicle_total [kg m2] : Constant  Value=Jzz  SampleTime=CSSampleTime
  km|h to m|s : Gain  Gain=1/3.6
  m_vehicle_total_[kg] : Constant  Value=mass  SampleTime=CSSampleTime
  s_Preview_LatCtrl : Subsystem
  wheel_base [m] : Constant  Value=length_l  SampleTime=CSSampleTime
  Actor/Traj_distance [m] : Outport
  Actor/Traj_angle [deg] : Outport  Port=2
  delta_steerwheel [deg] : Outport  Port=3
  wires:
  km|h to m|s/1 -> Calculate delta steering error/2(In2), s_Preview_LatCtrl/2(v_x_Vehicle_Min[m|s])
  Gain/1 -> Mux/3
  Mux/1 -> CTRL REFERENCES/3(TrajOffset [m,m,rad])
  ActorOffset_Left(+) / Right(-) [m]/1 -> CTRL REFERENCES/4(ActorOffset_Left(+) / Right(-)_[m])
  Demux/1 -> Mux/1
  Demux/2 -> Mux/2
  Demux/3 -> Gain/1
  TrajOffset x,y,Y [m,m,deg]/1 -> Demux/1
  CTRL REFERENCES/2(Actor/Traj_angle [deg]) -> Actor/Traj_angle [deg]/1
  CTRL REFERENCES/1(Actor/Traj_distance [m]) -> Actor/Traj_distance [m]/1
  Calculate delta steering error/1(Out1) -> SteeringWheelAngle/1(Angle_Steering[rad])
  vx [m/s]/1 -> Memory1/1
  vy [m/s]/1 -> Memory2/1
  CorneringStiffness_Tyres_Front [N/rad]/1 -> Calculate delta steering error/6(In6)
  m_vehicle_total_[kg]/1 -> Calculate delta steering error/8(In8)
  inertia_z_vehicle_total [kg m2]/1 -> Calculate delta steering error/9(In9)
  steering_ratio[-]/1 -> SteeringWheelAngle/2(i_Steering[])
  SteeringWheelAngle/1(Angle_SteeringWheel[deg]) -> Gain4/1, Memory/1
  Memory/1 -> SteeringWheelAngle/3(Angle_SteeringWheel_Last[deg])
  Constant6/1 -> SteeringWheelAngle/4(LatCtrl1_Enable[0Off|1On])
  Avoid_0/1 -> Calculate delta steering error/3(In3), s_Preview_LatCtrl/3(t_Preview_LatCtrl[s])
  Const_v_x_Vehicle_Min[km|h]/1 -> km|h to m|s/1
  s_Preview_LatCtrl/1(s_Preview_LatCtrl[m]) -> CTRL REFERENCES/2(Position Preview Distance [m])
  Const_t_Preview_LatCtrl[s]/1 -> Avoid_0/1
  Gain4/1 -> delta_steerwheel [deg]/1
  Distance_frontaxle_COG(+) [m]/1 -> Calculate delta steering error/11(In11)
  CorneringStiffness_Tyres_Rear [N/rad]/1 -> Calculate delta steering error/7(In7)
  Yaw rate [deg/s]/1 -> deg to rad/1
  deg to rad/1 -> Calculate delta steering error/5(In5)
  Gain1/1 -> Mux1/3
  Demux1/1 -> Mux1/1
  Demux1/2 -> Mux1/2
  Demux1/3 -> Gain1/1
  position x,y,Y [m,m,deg]/1 -> Demux1/1
  Mux1/1 -> CTRL REFERENCES/1(Pos x,y,Y [m,m,rad])
  wheel_base [m]/1 -> Calculate delta steering error/12(In12)
  CTRL REFERENCES/3(e_Lat [m]) -> Calculate delta steering error/10(In10)
  Memory1/1 -> Calculate delta steering error/1(In1), s_Preview_LatCtrl/1(v_x_Vehicle[m|s])
  Memory2/1 -> Calculate delta steering error/4(In4)

== system testemplanner_cs/Audi_A8_Sedan_2/PathFollower_Preview_1/LongitudinalController ==
  v_actual [m/s] : Inport
  Desired Velocity [m/s] : Inport  Port=2
  Initial Velocity [m/s] : Inport  Port=3
  Check_Initial_Velocity : Subsystem
  Demux : Demux  Outputs=3
  GearNormal : Constant
  "GearNormal " : Constant
  If Desired Velocity = 0 : Subsystem  TreatAsAtomicUnit=on
  If Desired Velocity ~= 0 : Subsystem  TreatAsAtomicUnit=on
  Memory External IC : Subsystem
  Merge : Merge
  Mux : Mux  Inputs=3
  Mux2 : Mux  Inputs=3
  Sum4 : Sum  Inputs=|+-
  if : If  IfExpression=u1 == 0  SampleTime=CSSampleTime
  throttle [%] : Outport
  brake pressure [bar] : Outport  Port=2
  v0 [m/s] : Outport  Port=3
  Auto_GearShift : Outport  Port=4
  wires:
  v_actual [m/s]/1 -> Check_Initial_Velocity/1(" v_actual_[m|s]"), Memory External IC/1(u)
  Memory External IC/1(y) -> Sum4/2
  Sum4/1 -> If Desired Velocity ~= 0/2(Desired Velocity [m/s])
  Desired Velocity [m/s]/1 -> if/1, Sum4/1
  Initial Velocity [m/s]/1 -> Check_Initial_Velocity/2(Initial_Velocity_[m|s]), Memory External IC/2(IC), v0 [m/s]/1
  GearNormal/1 -> If Desired Velocity = 0/1(In1)
  Merge/1 -> Demux/1
  If Desired Velocity = 0/1(throttle [%]) -> Mux/1
  If Desired Velocity = 0/2(brake pressure [bar]) -> Mux/2
  Mux2/1 -> Merge/2
  Mux/1 -> Merge/1
  Demux/1 -> throttle [%]/1
  Demux/2 -> brake pressure [bar]/1
  Demux/3 -> Auto_GearShift/1
  "GearNormal "/1 -> If Desired Velocity ~= 0/1(In1)
  If Desired Velocity = 0/3(Auto_GearShift) -> Mux/3
  if/2 -> If Desired Velocity ~= 0/Action
  if/1 -> If Desired Velocity = 0/Action
  If Desired Velocity ~= 0/1(throttle [%]) -> Mux2/1
  If Desired Velocity ~= 0/2(brake pressure [bar]) -> Mux2/2
  If Desired Velocity ~= 0/3(Auto_GearShift) -> Mux2/3

== system testemplanner_cs/Audi_A8_Sedan_2/SELF_Demux/compas converter ==
  rotz [rad] : Inport
  cart2compas : Subsystem
  rad2deg : Gain  Gain=180/pi
  heading [deg] : Outport
  wires:
  rad2deg/1 -> cart2compas/1(Angle [deg])
  rotz [rad]/1 -> rad2deg/1
  cart2compas/1(heading [deg]) -> heading [deg]/1
